simulink model "RI_EG_ISZM"  (R2013b)
settings: Solver=ode45  StartTime=0.0  StopTime=25e-3  RelTol=1e-3
libraries: RI_MK x2
settings Model: Creator=Szalay  LastModifiedBy=Szalay

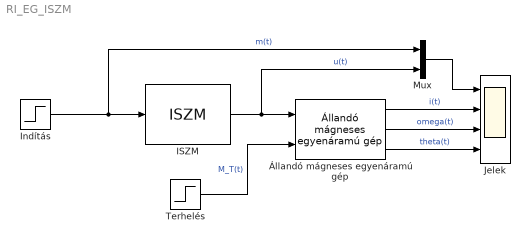
== system RI_EG_ISZM ==
  ISZM : RI_MK/ISZM  U_T=48  f_ISZM=25000  T_S=100e-9
  Indítás : Step  Time=1e-3  After=12  SampleTime=0
  Jelek : Scope  NumInputPorts=4
      settings: ShowLegends=on  YMin=-5~-5~-5~-5  YMax=5~5~5~5
  Mux : Mux  Inputs=2
  Terhelés : Step  Time=15e-3  After=0.1  SampleTime=0
  Állandó mágneses egyenáramú gép : RI_MK/Állandó mágneses egyenáramú gép  R=1.76  L=658e-6  k_T=68.3e-3  k_E=68.3e-3  J=99.5e-7  B=5.7301e-06  i_0=0  omega_0=0  theta_0=0
  wires:
  ISZM/1 -> Mux/2, Állandó mágneses egyenáramú gép/1  "u(t)"
  Indítás/1 -> Mux/1, ISZM/1  "m(t)"
  Terhelés/1 -> Állandó mágneses egyenáramú gép/2  "M_T(t)"
  Állandó mágneses egyenáramú gép/1 -> Jelek/2  "i(t)"
  Állandó mágneses egyenáramú gép/2 -> Jelek/3  "omega(t)"
  Állandó mágneses egyenáramú gép/3 -> Jelek/4  "theta(t)"
  Mux/1 -> Jelek/1
